simulink model "sobel_filter"  (R2026a)
settings: Solver=VariableStepAuto
settings Model: Creator=svvb7  LastModifiedBy=svvb7

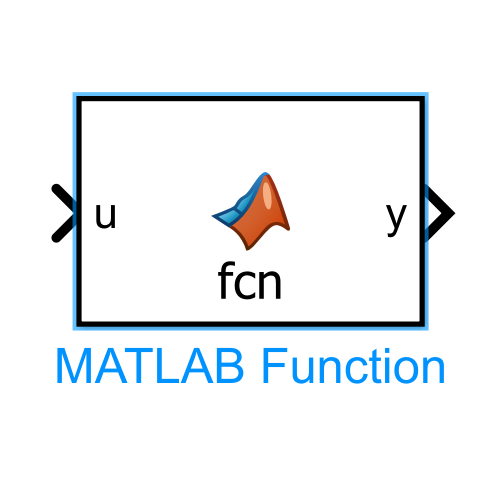
[thumbnail: Simulink's stored preview of the top-level diagram]
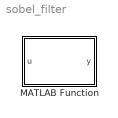
== system sobel_filter ==
  MATLAB Function : MATLAB Function  TreatAsAtomicUnit=on

== matlab function sobel_filter/MATLAB Function ==
  data: u input; y output
function y = fcn(u)
clc;
clear;
close all;

model = 'sobel_filter';

new_system(model);

open_system(model);

% Input
add_block('simulink/Sources/In1', ...
    [model '/Pixel_Input']);

% Sobel operation
add_block('simulink/Math Operations/Subtract', ...
    [model '/Gradient']);

% Output
add_block('simulink/Sinks/Out1', ...
    [model '/Edge_Output']);

% Connections
add_line(model,'Pixel_Input/1','Gradient/1');

add_line(model,'Gradient/1','Edge_Output/1');

save_system(model);

open_system(model);
